simulink model "test_model_sim"  (R2023a)
settings: Solver=ode4  StartTime=0.0  StopTime=40  FixedStep=0.01  RelTol=1e-3
values from neighbouring files (symbols this model uses):
  Ka = 4.5    [test_model_params.m]
  Kdc = 1.1    [test_model_params.m]
  Ki = 14.3    [test_model_params.m]
  Kr = -0.37    [test_model_params.m]
  l_M0 = 80*d2r    (= 1.3962634016)    [test_model_params.m]
  l_T0 = -45*d2r    (= -0.785398163397)    [test_model_params.m]
  V_T = 400    [test_model_params.m]
  X_M0 = 2000    [test_model_params.m]
  X_T0 = 100    [test_model_params.m]
  Z_M0 = 0    [test_model_params.m]
  Z_T0 = 20000    [test_model_params.m]
libraries: simulink x1
settings Model: Creator=acey4  LastModifiedBy=acey4

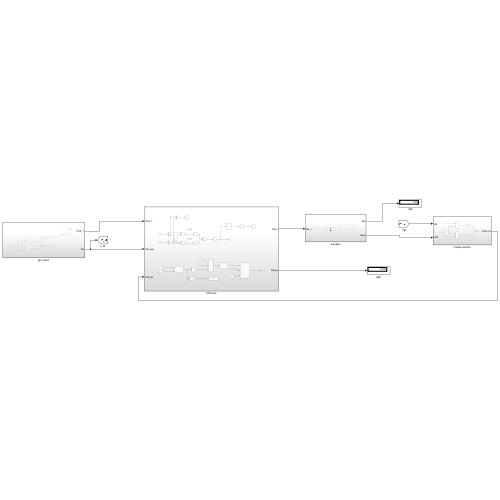
[thumbnail: Simulink's stored preview of the top-level diagram]
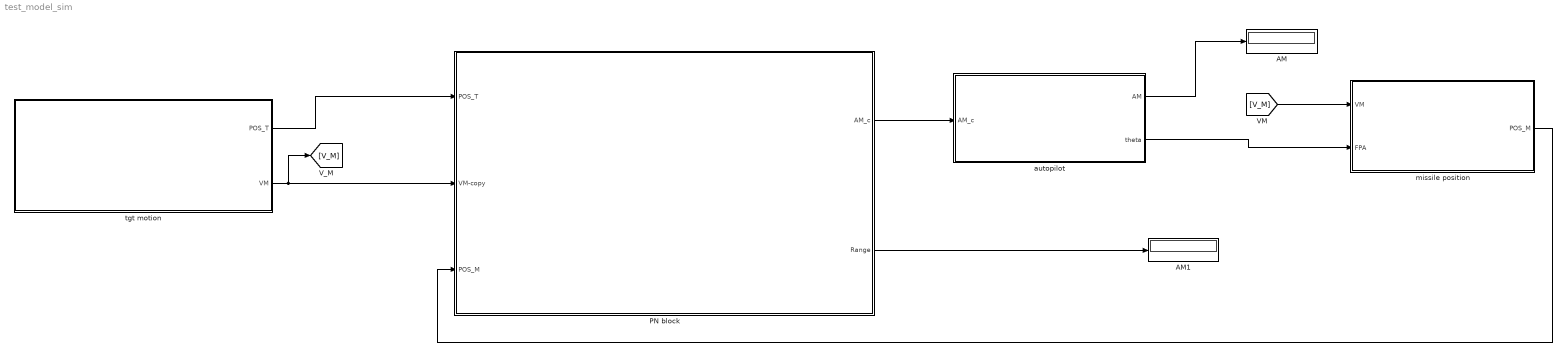
== system test_model_sim ==
  AM : Display
      settings: Format=bank
  AM1 : Display
      settings: Format=bank
  PN block : Subsystem
  autopilot : Subsystem
  missile position : Subsystem
  tgt motion : Subsystem
  wires:
  tgt motion/2(VM) -> [V_M], PN block/2(VM-copy)
  tgt motion/1(POS_T) -> PN block/1(POS_T)
  [V_M] -> missile position/1(VM)
  missile position/1(POS_M) -> PN block/3(POS_M)
  PN block/1(AM_c) -> autopilot/1(AM_c)
  autopilot/1(AM) -> AM/1
  PN block/2(Range) -> AM1/1
  autopilot/2(theta) -> missile position/2(FPA)

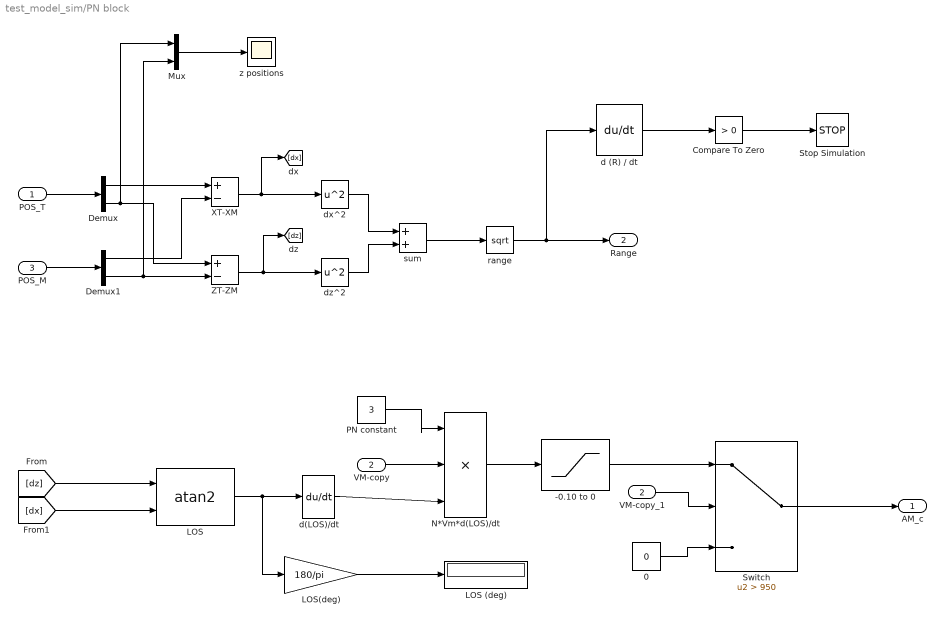
== system test_model_sim/PN block ==
  POS_T : Inport
  VM-copy : Inport  Port=2
  POS_M : Inport  Port=3
  -0.10 to 0 : Saturate  UpperLimit=0  LowerLimit=-0.10
  0 : Constant  Value=0
  Compare To Zero : simulink/Logic and Bit Operations/Compare To Zero  relop=>  OutDataTypeStr=boolean
  Demux : Demux  Outputs=2
  Demux1 : Demux  Outputs=2
  LOS : Trigonometry  Operator=atan2
  LOS (deg) : Display
  LOS(deg) : Gain  Gain=180/pi
  Mux : Mux  Inputs=2
  N*Vm*d(LOS)/dt : Product  Inputs=3
  PN constant : Constant  Value=3
  Stop Simulation : Stop
  Switch : Switch  Criteria=u2 > Threshold  Threshold=950  SaturateOnIntegerOverflow=off  InputSameDT=off
  VM-copy_1 : InportShadow  Port=2
  XT-XM : Sum  Inputs=+-
  ZT-ZM : Sum  Inputs=+-
  d (R) / dt : Derivative
  d(LOS)/dt : Derivative
  dx^2 : Math  Operator=square
  dz^2 : Math  Operator=square
  range : Sqrt
  sum : Sum
  z positions : Scope
  AM_c : Outport
  Range : Outport  Port=2
  wires:
  ZT-ZM/1 -> [dz], dz^2/1
  Compare To Zero/1 -> Stop Simulation/1
  XT-XM/1 -> [dx], dx^2/1
  POS_M/1 -> Demux1/1
  LOS/1 -> LOS(deg)/1, d(LOS)/dt/1
  Demux/1 -> XT-XM/1
  range/1 -> Range/1, d (R) / dt/1
  VM-copy/1 -> N*Vm*d(LOS)/dt/2
  Switch/1 -> AM_c/1
  -0.10 to 0/1 -> Switch/1
  Mux/1 -> z positions/1
  POS_T/1 -> Demux/1
  dz^2/1 -> sum/2
  LOS(deg)/1 -> LOS (deg)/1
  Demux1/2 -> Mux/2, ZT-ZM/2
  dx^2/1 -> sum/1
  d (R) / dt/1 -> Compare To Zero/1
  Demux/2 -> Mux/1, ZT-ZM/1
  Demux1/1 -> XT-XM/2
  N*Vm*d(LOS)/dt/1 -> -0.10 to 0/1
  d(LOS)/dt/1 -> N*Vm*d(LOS)/dt/3
  0/1 -> Switch/3
  [dz] -> LOS/1
  PN constant/1 -> N*Vm*d(LOS)/dt/1
  VM-copy_1/1 -> Switch/2
  [dx] -> LOS/2
  sum/1 -> range/1

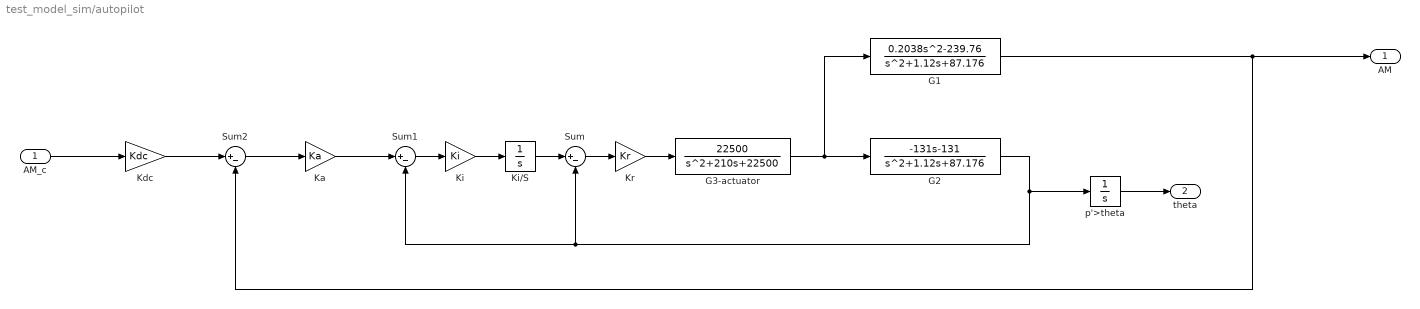
== system test_model_sim/autopilot ==
  AM_c : Inport
  G1 : TransferFcn  Numerator=[0.2038 0 -239.76]  Denominator=[1 1.12 87.176]
  G2 : TransferFcn  Numerator=[-131 -131]  Denominator=[1 1.12 87.176]
  G3-actuator : TransferFcn  Numerator=[22500]  Denominator=[1 210 22500]
  Ka : Gain  Gain=Ka
  Kdc : Gain  Gain=Kdc
  Ki : Gain  Gain=Ki
  Ki/S : Integrator
  Kr : Gain  Gain=Kr
  Sum : Sum  Inputs=|+-
  Sum1 : Sum  Inputs=|+-
  Sum2 : Sum  Inputs=|+-
  p'>theta : Integrator  InitialCondition=l_M0
  AM : Outport
  theta : Outport  Port=2
  wires:
  AM_c/1 -> Kdc/1
  G1/1 -> AM/1, Sum2/2
  Ki/1 -> Ki/S/1
  Sum/1 -> Kr/1
  Kdc/1 -> Sum2/1
  Ka/1 -> Sum1/1
  p'>theta/1 -> theta/1
  Kr/1 -> G3-actuator/1
  G2/1 -> p'>theta/1, Sum1/2, Sum/2
  G3-actuator/1 -> G1/1, G2/1
  Sum2/1 -> Ka/1
  Ki/S/1 -> Sum/1
  Sum1/1 -> Ki/1

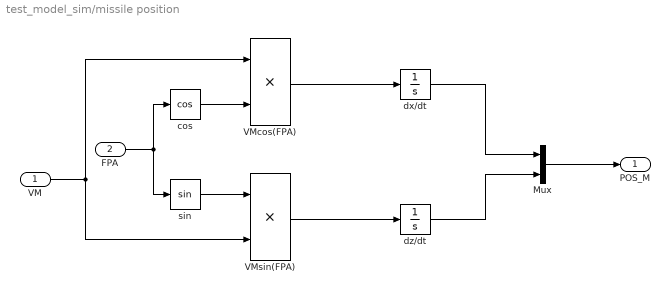
== system test_model_sim/missile position ==
  VM : Inport
  FPA : Inport  Port=2
  Mux : Mux  Inputs=2
  VMcos(FPA) : Product
  VMsin(FPA) : Product
  cos : Trigonometry  Operator=cos
  dx/dt : Integrator  InitialCondition=X_M0
  dz/dt : Integrator  InitialCondition=Z_M0
  sin : Trigonometry
  POS_M : Outport
  wires:
  cos/1 -> VMcos(FPA)/2
  VM/1 -> VMsin(FPA)/2, VMcos(FPA)/1
  dz/dt/1 -> Mux/2
  Mux/1 -> POS_M/1
  FPA/1 -> cos/1, sin/1
  VMsin(FPA)/1 -> dz/dt/1
  VMcos(FPA)/1 -> dx/dt/1
  sin/1 -> VMsin(FPA)/1
  dx/dt/1 -> Mux/1

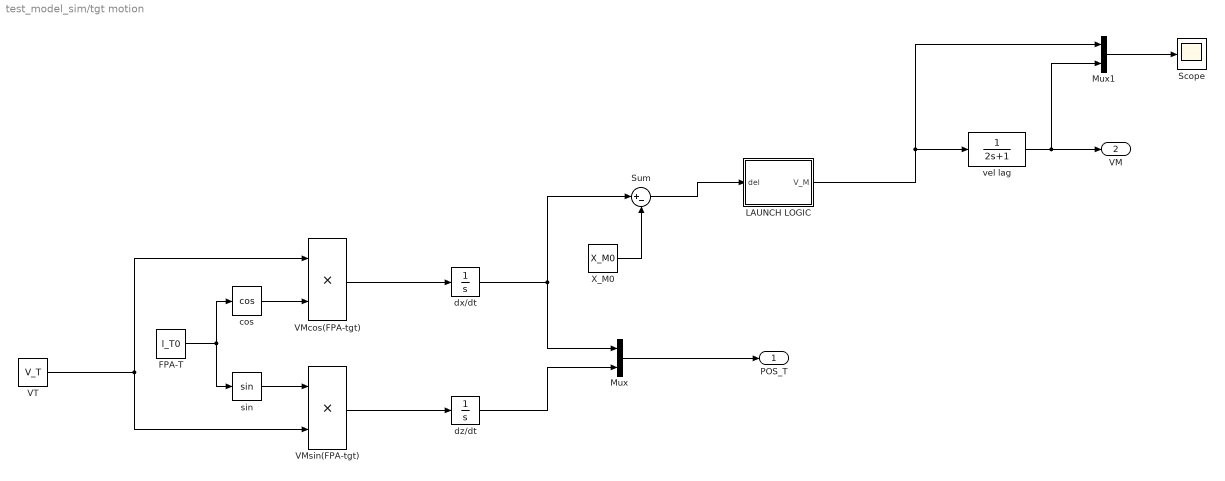
== system test_model_sim/tgt motion ==
  FPA-T : Constant  Value=l_T0
  LAUNCH LOGIC : MATLAB Function  TreatAsAtomicUnit=on
  Mux : Mux  Inputs=2
  Mux1 : Mux  Inputs=2
  Scope : Scope
  Sum : Sum  Inputs=|+-
  VMcos(FPA-tgt) : Product
  VMsin(FPA-tgt) : Product
  VT : Constant  Value=V_T
  X_M0 : Constant  Value=X_M0
  cos : Trigonometry  Operator=cos
  dx/dt : Integrator  InitialCondition=X_T0
  dz/dt : Integrator  InitialCondition=Z_T0
  sin : Trigonometry
  vel lag : TransferFcn  Denominator=[2 1]
  POS_T : Outport
  VM : Outport  Port=2
  wires:
  LAUNCH LOGIC/1(V_M) -> Mux1/1, vel lag/1
  cos/1 -> VMcos(FPA-tgt)/2
  Sum/1 -> LAUNCH LOGIC/1(del)
  FPA-T/1 -> cos/1, sin/1
  VT/1 -> VMsin(FPA-tgt)/2, VMcos(FPA-tgt)/1
  vel lag/1 -> VM/1, Mux1/2
  dx/dt/1 -> Sum/1, Mux/1
  VMcos(FPA-tgt)/1 -> dx/dt/1
  sin/1 -> VMsin(FPA-tgt)/1
  Mux/1 -> POS_T/1
  VMsin(FPA-tgt)/1 -> dz/dt/1
  X_M0/1 -> Sum/2
  dz/dt/1 -> Mux/2
  Mux1/1 -> Scope/1

== matlab function test_model_sim/tgt motion/LAUNCH LOGIC ==
  settings: updateMethod=DISCRETE
  data: del input; V_M output
function V_M = fcn(del)

persistent f
persistent Vel

if isempty (f)
    f = 0;
end
if isempty (Vel)
    Vel = 0;
end

if f == 0 && del > -200
    f = 1;
    Vel = 1021 %missile velocity
end

V_M = Vel;
